simulink subsystem "ss_controller_nomtracking"  (R2024b)
settings: Solver=VariableStepAuto  StartTime=0.0  StopTime=10.0  RelTol=1e-3
values from neighbouring files (symbols this model uses):
  K_fb = lqry(sysG, 1, r)    [Controller_LAB3_LQR.m]    (also in Controller_LAB3_LQR_Matrix.m = lqr(sysG, Q, R))
undefined symbols (not defined in the file or in its folder): Nu, Nx, rpm2rads
settings Model: Creator=Utente  LastModifiedBy=Buton

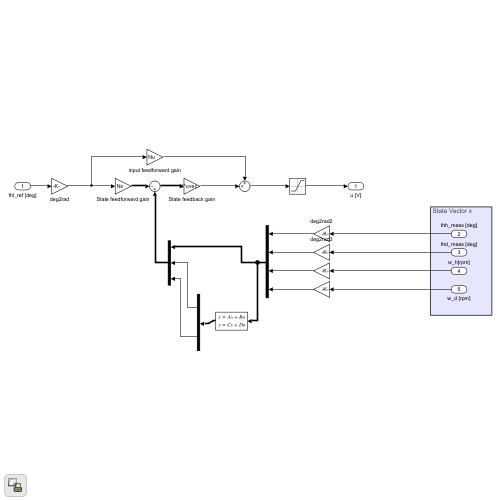
[thumbnail: Simulink's stored preview of the top-level diagram]
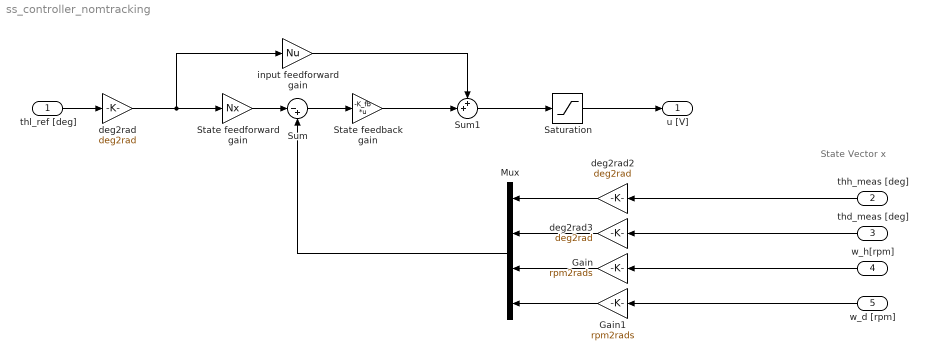
== system ss_controller_nomtracking ==
  note: State Vector x
  thl_ref [deg] : Inport
  thh_meas [deg] : Inport  Port=2
  thd_meas [deg] : Inport  Port=3
  w_h[rpm] : Inport  Port=4
  w_d [rpm] : Inport  Port=5
  Gain : Gain  Gain=rpm2rads
  Gain1 : Gain  Gain=rpm2rads
  Mux : Mux
  Saturation : Saturate  UpperLimit=12  LowerLimit=-12
  State feedback gain : Gain  Gain=-K_fb  Multiplication=Matrix(K*u) (u vector)
  State feedforward gain : Gain  Gain=Nx
  Sum : Sum  Inputs=|-+
  Sum1 : Sum  Inputs=++|
  deg2rad : Gain  Gain=deg2rad
  deg2rad2 : Gain  Gain=deg2rad
  deg2rad3 : Gain  Gain=deg2rad
  input feedforward gain : Gain  Gain=Nu
  u [V] : Outport
  wires:
  State feedforward gain/1 -> Sum/1
  Sum/1 -> State feedback gain/1
  Sum1/1 -> Saturation/1
  deg2rad/1 -> input feedforward gain/1, State feedforward gain/1
  thd_meas [deg]/1 -> deg2rad3/1
  State feedback gain/1 -> Sum1/2
  thl_ref [deg]/1 -> deg2rad/1
  input feedforward gain/1 -> Sum1/1
  Saturation/1 -> u [V]/1
  deg2rad2/1 -> Mux/1
  deg2rad3/1 -> Mux/2
  thh_meas [deg]/1 -> deg2rad2/1
  Gain/1 -> Mux/3
  w_h[rpm]/1 -> Gain/1
  w_d [rpm]/1 -> Gain1/1
  Gain1/1 -> Mux/4
  Mux/1 -> Sum/2
